simulink model "P"  (R2022a)
settings: Solver=VariableStepAuto  StartTime=0.0  StopTime=100  RelTol=1e-3
settings Model: Creator=ac133867  LastModifiedBy=cunis
settings DebuggingCC: UnconnectedInputMsg=warning  UnconnectedOutputMsg=warning  UnconnectedLineMsg=warning
settings RTWCC: DLArmComputeVersion=19.05

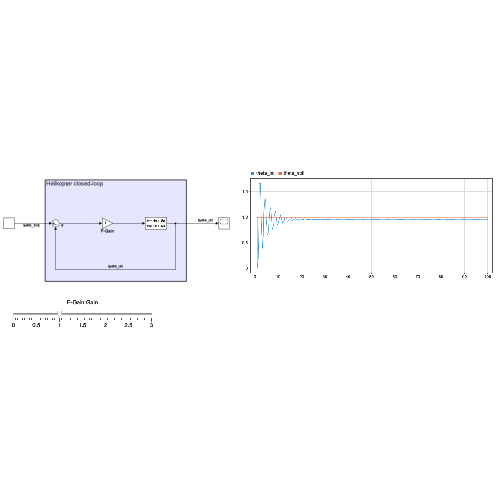
[thumbnail: Simulink's stored preview of the top-level diagram]
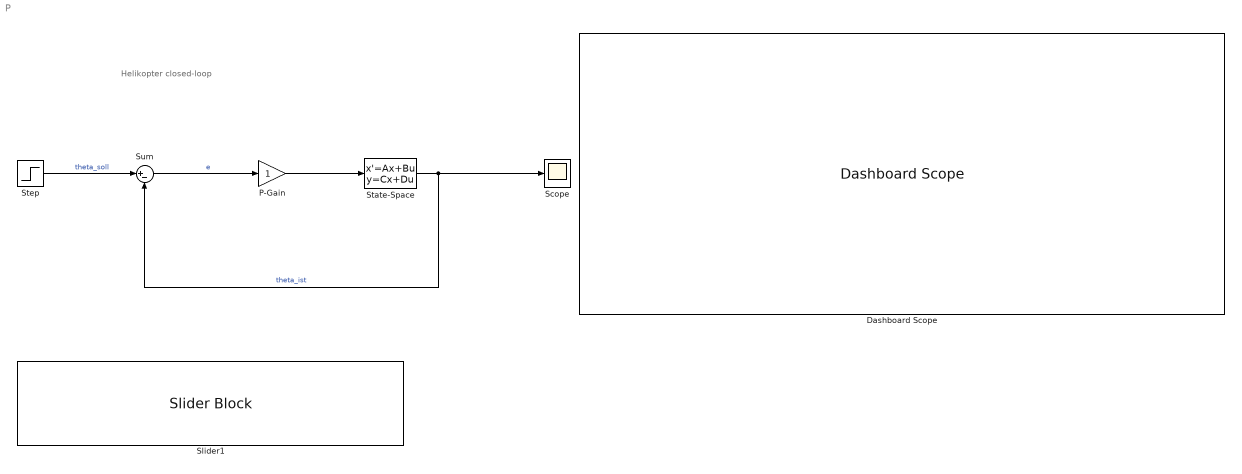
== system P ==
  note: Helikopter closed-loop
  Dashboard Scope : DashboardScope
  P-Gain : Gain
  Scope : Scope
  Slider1 : SliderBlock  ScaleMax=3  TickInterval=.5
  State-Space : StateSpace  A=[-0.2040 1.392 -9.8019; 0.0073 -0.4875 -0.0313; 0 1 0]  B=[-2.1242; 8.2631;0]  C=[0;0;1]'  D=0  InitialCondition=0
  Step : Step  SampleTime=0
  Sum : Sum  Inputs=|+-
  wires:
  Step/1 -> Sum/1  "theta_soll"
  P-Gain/1 -> State-Space/1
  Sum/1 -> P-Gain/1  "e"
  State-Space/1 -> Scope/1, Sum/2  "theta_ist"
